simulink model "realtime_controller"  (R2025b)
settings: Solver=FixedStepAuto  StartTime=0.0  StopTime=inf  FixedStep=0.01  MaxStep=0.0001  RelTol=1e-3
model workspace (MAT data in the model file):
  B = 3.5077e-06
  J = 3.2284e-06
  Kt = 0.0274
  L = 2.75e-06
  Px_LUT = [72.8945083618 76.6020507812 80.0916442871 83.3246154785 86.26612854 88.8862457275 91.1605911255 93.0707244873 94.6042098999 95.7543792725 96.5199050903 96.9042816162 96.9152145386 96.5639724731 95.8647842407 94.8342666626 93.4909515381 91.8547897339 89.9468231201 87.7888336182 85.4030838013 82.8120956421 80.0384292603 77.1045608521 74.0327148438 70.8447647095 67.5620803833 64.2054595947 60.7950210571 57.3501052856 53.8891906738 50.4297790527 46.9883308411 43.5801582336 40.2193336487 36.9186134338 33.6893348694 30.5413703918 27.483045578 24.5211086273 21.6607170105 18.9054584503 16.2574234009 13.7173147202 11.2846326828 8.95790672302 6.73498630524 4.61337375641 2.59057831764 0.664467632771 -1.16641640663 -2.90260267258 -4.54352331161 -6.08744049072 -7.53147363663 -8.87170600891 -10.1033649445 -11.22103405 -12.2188882828 -13.090924263 -13.8311738968 -14.4338855743 -14.8936719894 -15.2056322098 -15.3654279709 -15.3693389893 -15.2142906189 -14.8978567123 -14.4182472229 -13.7742786407 -12.9653301239 -11.9912958145 -10.8525152206 -9.54971599579 -8.08393192291 -6.45643568039 -4.66865777969 -2.72211909294 -0.61836206913 1.64110088348 4.05482435226 6.6214389801 9.33963012695 12.208067894 15.2252807617 18.3894691467 21.6982364655 25.1482276917 28.734703064 32.4510154724 36.2880249023 40.2335128784 44.2715797424 48.3821792603 52.5407600403 56.7181930542 60.8809700012 64.9917602539 69.0102767944 72.8945083618]
  Py_LUT = [145.51965332 149.831832886 154.01940918 158.062957764 161.947036743 165.659683228 169.191879272 172.536972046 175.689926147 178.646850586 181.404403687 183.959472656 186.308914185 188.44934082 190.377151489 192.088546753 193.57951355 194.84602356 195.884170532 196.690216064 197.260864258 197.593276978 197.685287476 197.535476685 197.143264771 196.509063721 195.634277344 194.521408081 193.174133301 191.597320557 189.797027588 187.78062439 185.556686401 183.135070801 180.526931763 177.74458313 174.801589966 171.712585449 168.493286133 165.160308838 161.731033325 158.223480225 154.655960083 151.046920776 147.414581299 143.776626587 140.149795532 136.549667358 132.990280151 129.483917236 126.041030884 122.670181274 119.378143311 116.170150757 113.050140381 110.021156311 107.085639954 104.245857239 101.504173279 98.8633117676 96.3265914917 93.8980255127 91.5824508667 89.3855133057 87.3137207031 85.3743896484 83.5755691528 81.925994873 80.4349822998 79.1123504639 77.9683151245 77.013381958 76.2582168579 75.7135772705 75.3901138306 75.2982940674 75.4482421875 75.8495407104 76.5110855103 77.4408798218 78.6457595825 80.1312026978 81.9009857178 83.9569168091 86.2984542847 88.922416687 91.8225784302 94.9893722534 98.4095993042 102.066230774 105.938323975 110.001068115 114.226104736 118.581939697 123.034675598 127.548919678 132.088790894 136.61907959 141.106292725 145.51965332]
  R = 4
  Ts = 0.01
  a = 1
  theta2_LUT = [0 0.0634665191174 0.126933038235 0.190399557352 0.253866076469 0.317332595587 0.380799114704 0.444265633821 0.507732152939 0.571198642254 0.634665191174 0.698131680489 0.761598229408 0.825064718723 0.888531267643 0.951997756958 1.01546430588 1.0789308548 1.14239728451 1.20586383343 1.26933038235 1.33279693127 1.39626336098 1.4597299099 1.52319645882 1.58666300774 1.65012943745 1.71359598637 1.77706253529 1.84052908421 1.90399551392 1.96746206284 2.03092861176 2.09439516068 2.15786170959 2.2213280201 2.28479456902 2.34826111794 2.41172766685 2.47519421577 2.53866076469 2.60212731361 2.66559386253 2.72906017303 2.79252672195 2.85599327087 2.91945981979 2.98292636871 3.04639291763 3.10985946655 3.17332601547 3.23679232597 3.30025887489 3.36372542381 3.42719197273 3.49065852165 3.55412507057 3.61759161949 3.68105816841 3.74452447891 3.80799102783 3.87145757675 3.93492412567 3.99839067459 4.06185722351 4.12532377243 4.18879032135 4.25225687027 4.31572341919 4.37918996811 4.44265604019 4.50612258911 4.56958913803 4.63305568695 4.69652223587 4.75998878479 4.82345533371 4.88692188263 4.95038843155 5.01385498047 5.07732152939 5.14078807831 5.20425462723 5.26772117615 5.33118772507 5.39465427399 5.45812034607 5.52158689499 5.58505344391 5.64851999283 5.71198654175 5.77545309067 5.83891963959 5.90238618851 5.96585273743 6.02931928635 6.09278583527 6.15625238419 6.21971893311 6.28318548203]
undefined symbols (not defined in the file or in its folder): ControlMode, f
libraries: svdutilitieslib x5, arduinolib x5, slpidlib x2, instrumentlib x2, simulink x1, arduinosensorlib x1
settings Model: ExtModeTrigDuration=2  Creator=msmca  LastModifiedBy=msmca
settings SolverCC: AutoInsertRateTranBlk=on
settings DataIOCC: ReturnWorkspaceOutputs=off
settings OptimizationCC: DefaultParameterBehavior=Inlined  EnhancedBackFolding=on  PassReuseOutputArgsAs=Individual arguments  ZeroExternalMemoryAtStartup=off  ZeroInternalMemoryAtStartup=off  MaxStackSize=64  OptimizeBlockOrder=speed  DifferentSizesBufferReuse=on  OptimizationCustomize=off  EfficientTunableParamExpr=on
settings DebuggingCC: ParameterTunabilityLossMsg=error
settings HardwareCC: ProdBitPerInt=16.0  ProdBitPerPointer=16.0  ProdBitPerSizeT=16.0  ProdBitPerPtrDiffT=16.0  ProdLargestAtomicFloat=None  ProdWordSize=8.0  ProdHWDeviceType=Atmel->AVR
settings SFSimCC: MATLABDynamicMemAlloc=off
settings RTWCC: SystemTargetFile=ert.tlc  HardwareBoard=Arduino Uno  TemplateMakefile=ert_default_tmf  Toolchain=Arduino AVR  BuildConfiguration=Faster Runs  Description=Embedded Coder
settings CodeAppCC: ForceParamTrailComments=on  IgnoreCustomStorageClasses=off  OperatorAnnotations=on  SimulinkDataObjDesc=on  SFDataObjDesc=on  InsertBlockDesc=on
settings ERTTargetCC: ExtModeTransport=3.0  ExtModeStaticAlloc=on  ExtModeAutomaticAllocSize=off  ExtModeStaticAllocSize=250.0  ExtModeMexFile=ext_xcp  ExtModeIntrfLevel=Level2 - Open  InlinedParameterPlacement=Hierarchical  SupportContinuousTime=on  SupportVariableSizeSignals=on

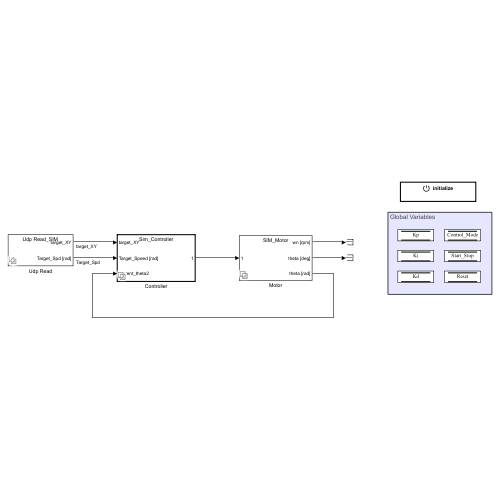
[thumbnail: Simulink's stored preview of the top-level diagram]
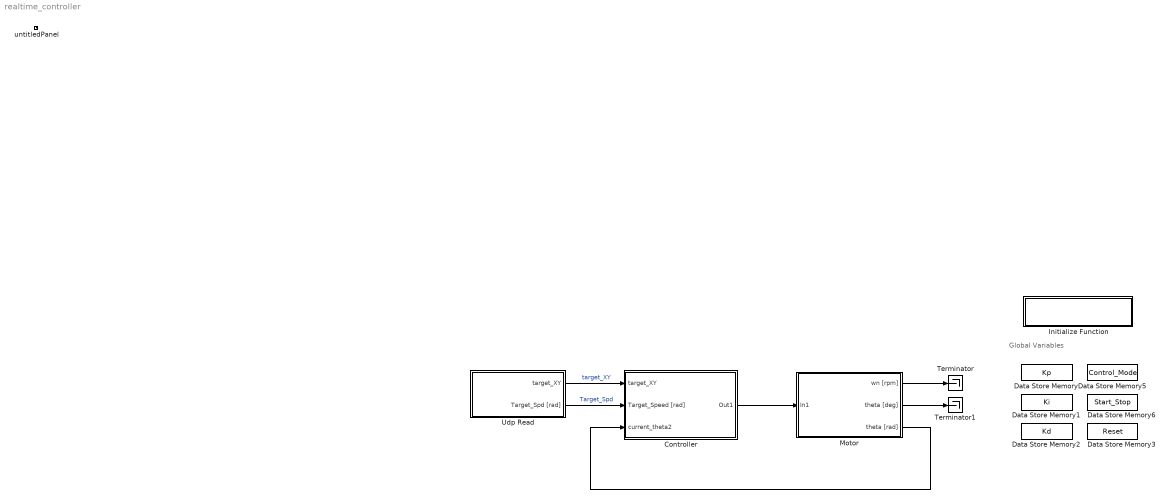
== system realtime_controller ==
  note: Global Variables
  Controller : Subsystem  TreatAsAtomicUnit=on  Variant=on  VariantControlMode=sim codegen switching  VariantControl=Controller  EmptyChoice=on
  Data Store Memory : DataStoreMemory  DataStoreName=Kp  WriteAfterWriteMsg=warning  ShowAdditionalParam=off
  Data Store Memory1 : DataStoreMemory  DataStoreName=Ki  WriteAfterWriteMsg=warning  ShowAdditionalParam=off
  Data Store Memory2 : DataStoreMemory  DataStoreName=Kd  WriteAfterWriteMsg=warning  ShowAdditionalParam=off
  Data Store Memory3 : DataStoreMemory  DataStoreName=Reset  WriteAfterWriteMsg=warning  ShowAdditionalParam=off
  Data Store Memory5 : DataStoreMemory  DataStoreName=Control_Mode  WriteAfterWriteMsg=warning  ShowAdditionalParam=off
  Data Store Memory6 : DataStoreMemory  DataStoreName=Start_Stop  WriteAfterWriteMsg=warning  ShowAdditionalParam=off  OutDataTypeStr=uint8
  Initialize Function : Subsystem  TreatAsAtomicUnit=on
  Motor : Subsystem  Variant=on  VariantControlMode=sim codegen switching  EmptyChoice=on
  Terminator : Terminator
  Terminator1 : Terminator
  Udp Read : Subsystem  Variant=on  VariantControlMode=sim codegen switching  EmptyChoice=on
  untitledPanel : Subsystem  Tag=HiddenForWebPanel  IsWebBlockPanel=on
  wires:
  Controller/1(Out1) -> Motor/1(In1)
  Motor/1(wn [rpm]) -> Terminator/1
  Motor/2(theta [deg]) -> Terminator1/1
  Motor/3(theta [rad]) -> Controller/3(current_theta2)
  Udp Read/1(target_XY) -> Controller/1(target_XY)  "target_XY"
  Udp Read/2(Target_Spd [rad]) -> Controller/2(Target_Speed [rad])  "Target_Spd"

== system realtime_controller/Controller ==
  target_XY : Inport
  Target_Speed [rad] : Inport  Port=2
  current_theta2 : Inport  Port=3
  Codegen_Controller : Subsystem  TreatAsAtomicUnit=on  VariantControl=(codegen)
  Sim_Controller : Subsystem  TreatAsAtomicUnit=on  VariantControl=(sim)
  Out1 : Outport

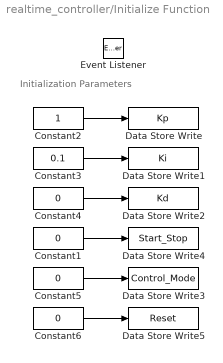
== system realtime_controller/Initialize Function ==
  note: Initialization Parameters
  Constant1 : Constant  Value=0  OutDataTypeStr=uint8
  Constant2 : Constant  OutDataTypeStr=single
  Constant3 : Constant  Value=0.1  OutDataTypeStr=single
  Constant4 : Constant  Value=0  OutDataTypeStr=single
  Constant5 : Constant  Value=0  OutDataTypeStr=uint8
  Constant6 : Constant  Value=0  OutDataTypeStr=uint8
  Data Store Write : DataStoreWrite  DataStoreName=Kp  IndexOptions=Index vector (dialog)  Indices=1  OutputSizes=1
  Data Store Write1 : DataStoreWrite  DataStoreName=Ki  IndexOptions=Index vector (dialog)  Indices=1  OutputSizes=1
  Data Store Write2 : DataStoreWrite  DataStoreName=Kd  IndexOptions=Index vector (dialog)  Indices=1  OutputSizes=1
  Data Store Write3 : DataStoreWrite  DataStoreName=Control_Mode  IndexOptions=Index vector (dialog)  Indices=1  OutputSizes=1
  Data Store Write4 : DataStoreWrite  DataStoreName=Start_Stop  IndexOptions=Index vector (dialog)  Indices=1  OutputSizes=1
  Data Store Write5 : DataStoreWrite  DataStoreName=Reset  IndexOptions=Index vector (dialog)  Indices=1  OutputSizes=1
  Event Listener : EventListener  DisableCoverage=on  EventName=reset
  wires:
  Constant2/1 -> Data Store Write/1
  Constant4/1 -> Data Store Write2/1
  Constant3/1 -> Data Store Write1/1
  Constant1/1 -> Data Store Write4/1
  Constant5/1 -> Data Store Write3/1
  Constant6/1 -> Data Store Write5/1

== system realtime_controller/Motor ==
  In1 : Inport
  Codgen_Motor : Subsystem  VariantControl=(codegen)
  SIM_Motor : Subsystem  VariantControl=(sim)
  wn [rpm] : Outport
  theta [deg] : Outport  Port=2
  theta [rad] : Outport  Port=3

== system realtime_controller/Udp Read ==
  Udp Read_Codegen : Subsystem  VariantControl=(codegen)
  Udp Read_SIM : Subsystem  VariantControl=(sim)
  target_XY : Outport
  Target_Spd [rad] : Outport  Port=2

== system realtime_controller/untitledPanel ==
  Display : DisplayBlock  Tag=HiddenForWebPanel  PanelInfo="{\"height\":69,\"left\":301,\"panelId\":\"panelId-5f5342a7-719f-4c1d-a791-b117091cac79\",\"top\":10,\"type\":\"panelChild\",\"version\":\"2019b\",\"width\":222,\"zIndex\":1500008}"  Transparency=1  GridColor=[0.502, 0.502, 0.502]
  Display1 : DisplayBlock  Tag=HiddenForWebPanel  PanelInfo="{\"height\":62,\"left\":196,\"panelId\":\"panelId-5f5342a7-719f-4c1d-a791-b117091cac79\",\"top\":15,\"type\":\"panelChild\",\"version\":\"2019b\",\"width\":94,\"zIndex\":1500004}"  Transparency=1  GridColor=[0.502, 0.502, 0.502]
  Display2 : DisplayBlock  Tag=HiddenForWebPanel  PanelInfo="{\"height\":57,\"left\":12,\"panelId\":\"panelId-5f5342a7-719f-4c1d-a791-b117091cac79\",\"top\":19,\"type\":\"panelChild\",\"version\":\"2019b\",\"width\":171,\"zIndex\":1500002}"  Format=Custom  Transparency=1  Layout=Fill available space  FormatString=%s  GridColor=[0.502, 0.502, 0.502]  ShowGrid=off
  Start/Stop : LampBlock  Tag=HiddenForWebPanel  PanelInfo="{\"height\":60,\"left\":550,\"panelId\":\"panelId-5f5342a7-719f-4c1d-a791-b117091cac79\",\"top\":20,\"type\":\"panelChild\",\"version\":\"2019b\",\"width\":65,\"zIndex\":1500006}"  DefaultColor=[192.0, 192.0, 192.0]
  panelInfo : PanelWebBlock  Tag=HiddenForWebPanel  PanelInfo="{\"compacted\":false,\"height\":86,\"isActiveTab\":true,\"left\":280,\"name\":\"Panel\",\"panelId\":\"panelId-5f5342a7-719f-4c1d-a791-b117091cac79\",\"tabIndex\":0,\"tabbedSetId\":\"tabbedSet4298033123\",\"top\":26,\"type\":\"panel\",\"version\":\"2019b\",\"visible\":true,\"width\":648,\"zIndex\":1500002}"  PanelSnapshot=<binary blob, 24248 chars, not shown>

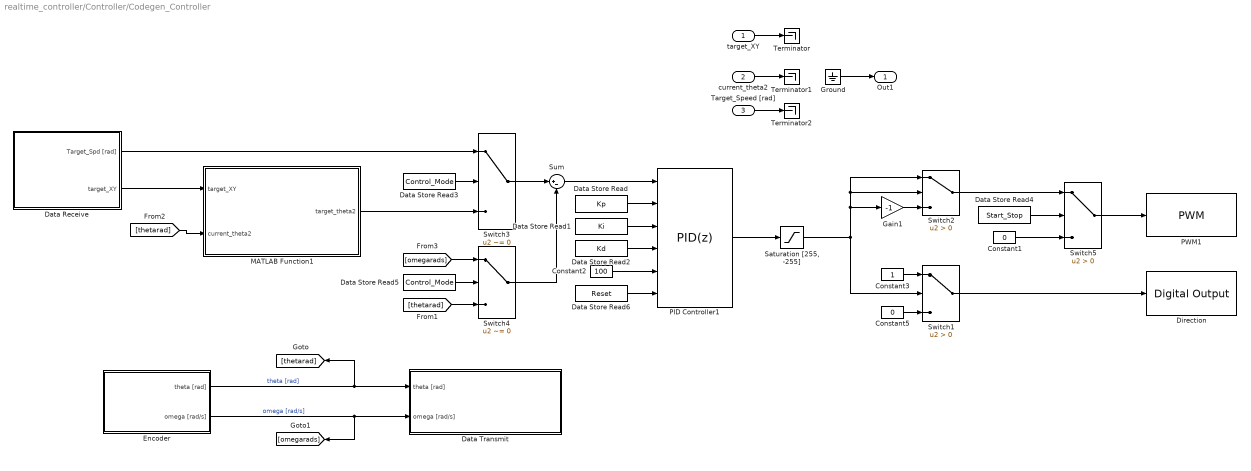
== system realtime_controller/Controller/Codegen_Controller ==
  target_XY : Inport
  current_theta2 : Inport  Port=2
  Target_Speed [rad] : Inport  Port=3
  Constant1 : Constant  Value=0  OutDataTypeStr=boolean
  Constant2 : Constant  Value=100  OutDataTypeStr=single
  Constant3 : Constant  OutDataTypeStr=boolean
  Constant5 : Constant  Value=0  OutDataTypeStr=boolean
  Data Receive : Subsystem
  Data Store Read : DataStoreRead  DataStoreName=Kp  IndexOptions=Index vector (dialog)  Indices=1  OutputSizes=1
  Data Store Read1 : DataStoreRead  DataStoreName=Ki  IndexOptions=Index vector (dialog)  Indices=1  OutputSizes=1
  Data Store Read2 : DataStoreRead  DataStoreName=Kd  IndexOptions=Index vector (dialog)  Indices=1  OutputSizes=1
  Data Store Read3 : DataStoreRead  DataStoreName=Control_Mode  IndexOptions=Index vector (dialog)  Indices=1  OutputSizes=1
  Data Store Read4 : DataStoreRead  DataStoreName=Start_Stop  IndexOptions=Index vector (dialog)  Indices=1  OutputSizes=1
  Data Store Read5 : DataStoreRead  DataStoreName=Control_Mode  IndexOptions=Index vector (dialog)  Indices=1  OutputSizes=1
  Data Store Read6 : DataStoreRead  DataStoreName=Reset  IndexOptions=Index vector (dialog)  Indices=1  OutputSizes=1
  Data Transmit : Subsystem
  Direction : arduinolib/Digital Output  pinNumber=9  Direction=output  blockPlatform=arduino
  Encoder : Subsystem
  Gain1 : Gain  Gain=-1
  Ground : Ground
  MATLAB Function1 : MATLAB Function  TreatAsAtomicUnit=on  VariantControl=CTRL_MODE == 1
      settings: RTWSystemCode=Inline
  PID Controller1 : slpidlib/PID Controller  Controller=PID  Form=Parallel  TimeDomain=Discrete-time  UseExternalTs=off  SampleTime=-1  IntegratorMethod=Forward Euler  FilterMethod=Forward Euler  ControllerParametersSource=external  P=236.110480401302  I=928.989984660749  UseKiTs=off  D=4.7957256427105  UseExternalDerivativeSource=off  N=1443.07789722776  UseFilter=on  TunerSelectOption=Transfer Function Based (PID Tuner App)  InitialConditionSource=internal  InitialConditionForIntegrator=0  InitialConditionForFilter=0  DifferentiatorICPrevScaledInput=0  ExternalReset=either  TrackingMode=off  Kt=1  LimitOutput=off  SatLimitsSource=internal  UpperSaturationLimit=24  LowerSaturationLimit=-24  LinearizeAsGain=on  AntiWindupMode=clamping  Kb=1  LimitIntegrator=on  UpperIntegratorSaturationLimit=35  LowerIntegratorSaturationLimit=-35  POutMin=[]  POutMax=[]  IOutMin=[]  IOutMax=[]  DOutMin=[]  DOutMax=[]  NOutMin=[]  NOutMax=[]  SumOutMin=[]  SumOutMax=[]  SaturationOutMin=[]  SaturationOutMax=[]  PParamMin=[]  PParamMax=[]  IParamMin=[]  IParamMax=[]  DParamMin=[]  DParamMax=[]  NParamMin=[]  NParamMax=[]  KbParamMin=[]  KbParamMax=[]  KtParamMin=[]  KtParamMax=[]  KbOutMin=[]  KbOutMax=[]  KtOutMin=[]  KtOutMax=[]  IntegratorOutMin=[]  IntegratorOutMax=[]  FilterOutMin=[]  FilterOutMax=[]  SumI1OutMin=[]  SumI1OutMax=[]  SumI2OutMin=[]  SumI2OutMax=[]  SumI3OutMin=[]  SumI3OutMax=[]  SumI4OutMin=[]  SumI4OutMax=[]  SumDOutMin=[]  SumDOutMax=[]  DifferentiatorOutMin=[]  DifferentiatorOutMax=[]  FilterDiffOutCoefMin=[]  FilterDiffOutCoefMax=[]  ReciprocalOutMin=[]  ReciprocalOutMax=[]  SumDenOutMin=[]  SumDenOutMax=[]  SumNumOutMin=[]  SumNumOutMax=[]  DivideOutMin=[]  DivideOutMax=[]  UdiffTsProdOutMin=[]  UdiffTsProdOutMax=[]  NTsProdOutMin=[]  NTsProdOutMax=[]  UintegralTsProdOutMin=[]  UintegralTsProdOutMax=[]  UngainTsProdOutMin=[]  UngainTsProdOutMax=[]  ClampingZeroOutDataTypeStr=Inherit: Inherit via back propagation  ClampingZeroOutMin=[]  ClampingZeroOutMax=[]  FilterDenConstantOutDataTypeStr=Inherit: Inherit via back propagation  FilterDenConstantOutMin=[]  FilterDenConstantOutMax=[]  PCopyOutDataTypeStr=Inherit: Inherit via back propagation  PCopyOutMin=[]  PCopyOutMax=[]  NCopyOutDataTypeStr=Inherit: Inherit via back propagation  NCopyOutMin=[]  NCopyOutMax=[]  IntegratorContinuousStateAttributes=''  IntegratorStateMustResolveToSignalObject=off  IntegratorRTWStateStorageClass=Auto  FilterContinuousStateAttributes=''  FilterStateMustResolveToSignalObject=off  FilterRTWStateStorageClass=Auto  ParallelPVariant=ExternalParameters  IdealPVariant=Disabled  IVariant=ExternalParameters  DVariant=ExternalParameters  IntegratorVariant=Discrete  SatVariant=Disabled  AWVariant=Passthrough  PCopyVariant=Disabled  TRVariant=Disabled  FdbkBlocksVariant=Forward  IdealPFdbkVariant=Disabled  SatFdbkVariant=Disabled  DerivativeFilterVariant=ForwardEulerFilter  NVariant=ExternalParameters  NCopyVariant=Disabled  FilterICVariant=InternalICsFilter  IntegratorICVariant=InternalICs  ExternalResetVariant=ExternalReset  TRSumVariant=Passthrough  SumFdbkVariant=Disabled  SumVariant=Sum_PID  TsampFilterVariant=InternalTs  TsampNgainVariant=Passthrough  TsampIntegralVariant=Disabled_SignalSpec  ExternalSaturationOutDataTypeStr=Inherit: Same as second input  DerivativeSourceVariant=ErrorSignal  PreIntVariant=InternalPreInt
  PWM1 : arduinolib/PWM  pinNumber=5  frequencyType=Default  desiredFrequency=490.2  achievableFrequency=490.2
  "Saturation [255, -255]" : Saturate  UpperLimit=254  LowerLimit=-254
  Sum : Sum  Inputs=|+-
  Switch1 : Switch  Criteria=u2 > Threshold  SaturateOnIntegerOverflow=off  InputSameDT=off
  Switch2 : Switch  Criteria=u2 > Threshold  OutDataTypeStr=single  SaturateOnIntegerOverflow=off  InputSameDT=off
  Switch3 : Switch  Criteria=u2 ~= 0  Threshold=0.5  SaturateOnIntegerOverflow=off  InputSameDT=off
  Switch4 : Switch  Criteria=u2 ~= 0  Threshold=0.5  SaturateOnIntegerOverflow=off  InputSameDT=off
  Switch5 : Switch  Criteria=u2 > Threshold  OutDataTypeStr=single  SaturateOnIntegerOverflow=off  InputSameDT=off
  Terminator : Terminator
  Terminator1 : Terminator
  Terminator2 : Terminator
  Out1 : Outport
  wires:
  PID Controller1/1 -> "Saturation [255, -255]"/1
  target_XY/1 -> Terminator/1
  current_theta2/1 -> Terminator1/1
  Data Receive/2(target_XY) -> MATLAB Function1/1(target_XY)
  Encoder/1(theta [rad]) -> Data Transmit/1(theta [rad]), [thetarad]  "theta [rad]"
  Encoder/2(omega [rad/s]) -> Data Transmit/2(omega [rad/s]), [omegarads]  "omega [rad/s]"
  Ground/1 -> Out1/1
  "Saturation [255, -255]"/1 -> Switch1/2, Gain1/1, Switch2/1, Switch2/2
  Gain1/1 -> Switch2/3
  Switch1/1 -> Direction/1
  Constant5/1 -> Switch1/3
  Constant3/1 -> Switch1/1
  Switch3/1 -> Sum/1
  Data Store Read3/1 -> Switch3/2
  MATLAB Function1/1(target_theta2) -> Switch3/3
  Switch4/1 -> Sum/2
  Data Store Read5/1 -> Switch4/2
  [thetarad] -> MATLAB Function1/2(current_theta2)
  [thetarad] -> Switch4/3
  [omegarads] -> Switch4/1
  Data Receive/1(Target_Spd [rad]) -> Switch3/1
  Switch5/1 -> PWM1/1
  Data Store Read4/1 -> Switch5/2
  Switch2/1 -> Switch5/1
  Constant1/1 -> Switch5/3
  Target_Speed [rad]/1 -> Terminator2/1
  Data Store Read/1 -> PID Controller1/2
  Data Store Read6/1 -> PID Controller1/6
  Data Store Read2/1 -> PID Controller1/4
  Data Store Read1/1 -> PID Controller1/3
  Sum/1 -> PID Controller1/1
  Constant2/1 -> PID Controller1/5

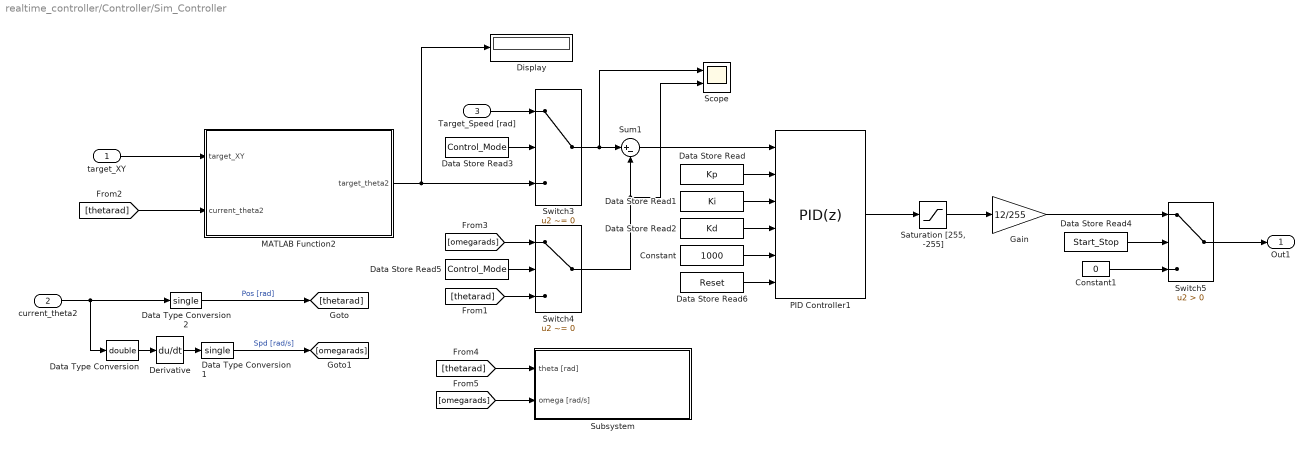
== system realtime_controller/Controller/Sim_Controller ==
  target_XY : Inport
  current_theta2 : Inport  Port=2
  Target_Speed [rad] : Inport  Port=3
  Constant : Constant  Value=1000  OutDataTypeStr=single
  Constant1 : Constant  Value=0  OutDataTypeStr=boolean
  Data Store Read : DataStoreRead  DataStoreName=Kp  IndexOptions=Index vector (dialog)  Indices=1  OutputSizes=1
  Data Store Read1 : DataStoreRead  DataStoreName=Ki  IndexOptions=Index vector (dialog)  Indices=1  OutputSizes=1
  Data Store Read2 : DataStoreRead  DataStoreName=Kd  IndexOptions=Index vector (dialog)  Indices=1  OutputSizes=1
  Data Store Read3 : DataStoreRead  DataStoreName=Control_Mode  IndexOptions=Index vector (dialog)  Indices=1  OutputSizes=1
  Data Store Read4 : DataStoreRead  DataStoreName=Start_Stop  IndexOptions=Index vector (dialog)  Indices=1  OutputSizes=1
  Data Store Read5 : DataStoreRead  DataStoreName=Control_Mode  IndexOptions=Index vector (dialog)  Indices=1  OutputSizes=1
  Data Store Read6 : DataStoreRead  DataStoreName=Reset  IndexOptions=Index vector (dialog)  Indices=1  OutputSizes=1
  Data Type Conversion : DataTypeConversion  OutDataTypeStr=double  SaturateOnIntegerOverflow=off  RndMeth=Floor
  Data Type Conversion1 : DataTypeConversion  OutDataTypeStr=single  SaturateOnIntegerOverflow=off  RndMeth=Floor
  Data Type Conversion2 : DataTypeConversion  OutDataTypeStr=single  SaturateOnIntegerOverflow=off  RndMeth=Floor
  Derivative : Derivative
  Display : Display
  Gain : Gain  Gain=12/255
  MATLAB Function2 : MATLAB Function  TreatAsAtomicUnit=on  VariantControl=CTRL_MODE == 1
  PID Controller1 : slpidlib/PID Controller  Controller=PID  Form=Parallel  TimeDomain=Discrete-time  UseExternalTs=off  SampleTime=-1  IntegratorMethod=Forward Euler  FilterMethod=Forward Euler  ControllerParametersSource=external  P=236.110480401302  I=928.989984660749  UseKiTs=off  D=4.7957256427105  UseExternalDerivativeSource=off  N=1443.07789722776  UseFilter=on  TunerSelectOption=Transfer Function Based (PID Tuner App)  InitialConditionSource=internal  InitialConditionForIntegrator=0  InitialConditionForFilter=0  DifferentiatorICPrevScaledInput=0  ExternalReset=either  TrackingMode=off  Kt=1  LimitOutput=off  SatLimitsSource=internal  UpperSaturationLimit=24  LowerSaturationLimit=-24  LinearizeAsGain=on  AntiWindupMode=clamping  Kb=1  LimitIntegrator=on  UpperIntegratorSaturationLimit=12  LowerIntegratorSaturationLimit=-12  POutMin=[]  POutMax=[]  IOutMin=[]  IOutMax=[]  DOutMin=[]  DOutMax=[]  NOutMin=[]  NOutMax=[]  SumOutMin=[]  SumOutMax=[]  SaturationOutMin=[]  SaturationOutMax=[]  PParamMin=[]  PParamMax=[]  IParamMin=[]  IParamMax=[]  DParamMin=[]  DParamMax=[]  NParamMin=[]  NParamMax=[]  KbParamMin=[]  KbParamMax=[]  KtParamMin=[]  KtParamMax=[]  KbOutMin=[]  KbOutMax=[]  KtOutMin=[]  KtOutMax=[]  IntegratorOutMin=[]  IntegratorOutMax=[]  FilterOutMin=[]  FilterOutMax=[]  SumI1OutMin=[]  SumI1OutMax=[]  SumI2OutMin=[]  SumI2OutMax=[]  SumI3OutMin=[]  SumI3OutMax=[]  SumI4OutMin=[]  SumI4OutMax=[]  SumDOutMin=[]  SumDOutMax=[]  DifferentiatorOutMin=[]  DifferentiatorOutMax=[]  FilterDiffOutCoefMin=[]  FilterDiffOutCoefMax=[]  ReciprocalOutMin=[]  ReciprocalOutMax=[]  SumDenOutMin=[]  SumDenOutMax=[]  SumNumOutMin=[]  SumNumOutMax=[]  DivideOutMin=[]  DivideOutMax=[]  UdiffTsProdOutMin=[]  UdiffTsProdOutMax=[]  NTsProdOutMin=[]  NTsProdOutMax=[]  UintegralTsProdOutMin=[]  UintegralTsProdOutMax=[]  UngainTsProdOutMin=[]  UngainTsProdOutMax=[]  ClampingZeroOutDataTypeStr=Inherit: Inherit via back propagation  ClampingZeroOutMin=[]  ClampingZeroOutMax=[]  FilterDenConstantOutDataTypeStr=Inherit: Inherit via back propagation  FilterDenConstantOutMin=[]  FilterDenConstantOutMax=[]  PCopyOutDataTypeStr=Inherit: Inherit via back propagation  PCopyOutMin=[]  PCopyOutMax=[]  NCopyOutDataTypeStr=Inherit: Inherit via back propagation  NCopyOutMin=[]  NCopyOutMax=[]  IntegratorContinuousStateAttributes=''  IntegratorStateMustResolveToSignalObject=off  IntegratorRTWStateStorageClass=Auto  FilterContinuousStateAttributes=''  FilterStateMustResolveToSignalObject=off  FilterRTWStateStorageClass=Auto  ParallelPVariant=ExternalParameters  IdealPVariant=Disabled  IVariant=ExternalParameters  DVariant=ExternalParameters  IntegratorVariant=Discrete  SatVariant=Disabled  AWVariant=Passthrough  PCopyVariant=Disabled  TRVariant=Disabled  FdbkBlocksVariant=Forward  IdealPFdbkVariant=Disabled  SatFdbkVariant=Disabled  DerivativeFilterVariant=ForwardEulerFilter  NVariant=ExternalParameters  NCopyVariant=Disabled  FilterICVariant=InternalICsFilter  IntegratorICVariant=InternalICs  ExternalResetVariant=ExternalReset  TRSumVariant=Passthrough  SumFdbkVariant=Disabled  SumVariant=Sum_PID  TsampFilterVariant=InternalTs  TsampNgainVariant=Passthrough  TsampIntegralVariant=Disabled_SignalSpec  ExternalSaturationOutDataTypeStr=Inherit: Same as second input  DerivativeSourceVariant=ErrorSignal  PreIntVariant=InternalPreInt
  "Saturation [255, -255]" : Saturate  UpperLimit=255  LowerLimit=-255
  Scope : Scope  NumInputPorts=2
      settings: ActiveDisplayYMinimum=-26.442962050437924  ActiveDisplayYMaximum=185.34457051753998
  Subsystem : Subsystem
  Sum1 : Sum  Inputs=|+-
  Switch3 : Switch  Criteria=u2 ~= 0  Threshold=0.5  SaturateOnIntegerOverflow=off  InputSameDT=off
  Switch4 : Switch  Criteria=u2 ~= 0  Threshold=0.5  SaturateOnIntegerOverflow=off  InputSameDT=off
  Switch5 : Switch  Criteria=u2 > Threshold  OutDataTypeStr=single  SaturateOnIntegerOverflow=off  InputSameDT=off
  Out1 : Outport
  wires:
  Data Store Read5/1 -> Switch4/2
  "Saturation [255, -255]"/1 -> Gain/1
  Data Store Read4/1 -> Switch5/2
  [thetarad] -> MATLAB Function2/2(current_theta2)
  Constant1/1 -> Switch5/3
  Data Store Read3/1 -> Switch3/2
  [omegarads] -> Switch4/1
  [thetarad] -> Switch4/3
  PID Controller1/1 -> "Saturation [255, -255]"/1
  Switch3/1 -> Scope/1, Sum1/1
  Switch4/1 -> Scope/2, Sum1/2
  Sum1/1 -> PID Controller1/1
  Switch5/1 -> Out1/1
  Gain/1 -> Switch5/1
  current_theta2/1 -> Data Type Conversion2/1, Data Type Conversion/1
  Derivative/1 -> Data Type Conversion1/1
  [thetarad] -> Subsystem/1(theta [rad])
  [omegarads] -> Subsystem/2(omega [rad/s])
  Data Type Conversion/1 -> Derivative/1
  Data Type Conversion1/1 -> [omegarads]  "Spd [rad/s]"
  MATLAB Function2/1(target_theta2) -> Display/1, Switch3/3
  Data Store Read/1 -> PID Controller1/2
  Data Store Read2/1 -> PID Controller1/4
  Constant/1 -> PID Controller1/5
  Data Type Conversion2/1 -> [thetarad]  "Pos [rad]"
  Target_Speed [rad]/1 -> Switch3/1
  target_XY/1 -> MATLAB Function2/1(target_XY)
  Data Store Read1/1 -> PID Controller1/3
  Data Store Read6/1 -> PID Controller1/6

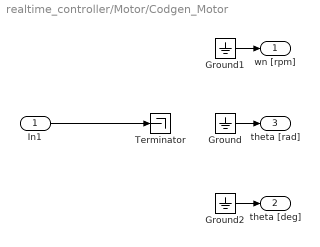
== system realtime_controller/Motor/Codgen_Motor ==
  In1 : Inport  OutDataTypeStr=single
  Ground : Ground
  Ground1 : Ground
  Ground2 : Ground
  Terminator : Terminator
  wn [rpm] : Outport  OutDataTypeStr=single
  theta [deg] : Outport  Port=2  OutDataTypeStr=single
  theta [rad] : Outport  Port=3  OutDataTypeStr=single
  wires:
  In1/1 -> Terminator/1
  Ground/1 -> theta [rad]/1
  Ground1/1 -> wn [rpm]/1
  Ground2/1 -> theta [deg]/1

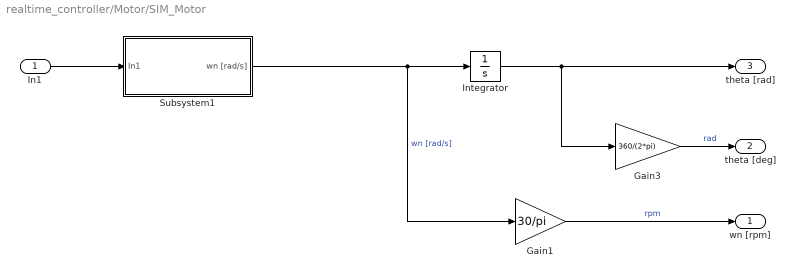
== system realtime_controller/Motor/SIM_Motor ==
  In1 : Inport
  Gain1 : Gain  Gain=30/pi  OutDataTypeStr=single
  Gain3 : Gain  Gain=360/(2*pi)  OutDataTypeStr=single
  Integrator : Integrator
  Subsystem1 : Subsystem
  wn [rpm] : Outport
  theta [deg] : Outport  Port=2
  theta [rad] : Outport  Port=3
  wires:
  Gain3/1 -> theta [deg]/1  "rad"
  Gain1/1 -> wn [rpm]/1  "rpm"
  In1/1 -> Subsystem1/1(In1)
  Integrator/1 -> theta [rad]/1, Gain3/1
  Subsystem1/1(wn [rad/s]) -> Integrator/1, Gain1/1  "wn [rad/s]"

== system realtime_controller/Udp Read/Udp Read_Codegen ==
  Ground : Ground
  Ground1 : Ground
  target_XY : Outport  OutDataTypeStr=single
  Target_Spd [rad] : Outport  Port=2  OutDataTypeStr=single
  wires:
  Ground/1 -> target_XY/1
  Ground1/1 -> Target_Spd [rad]/1

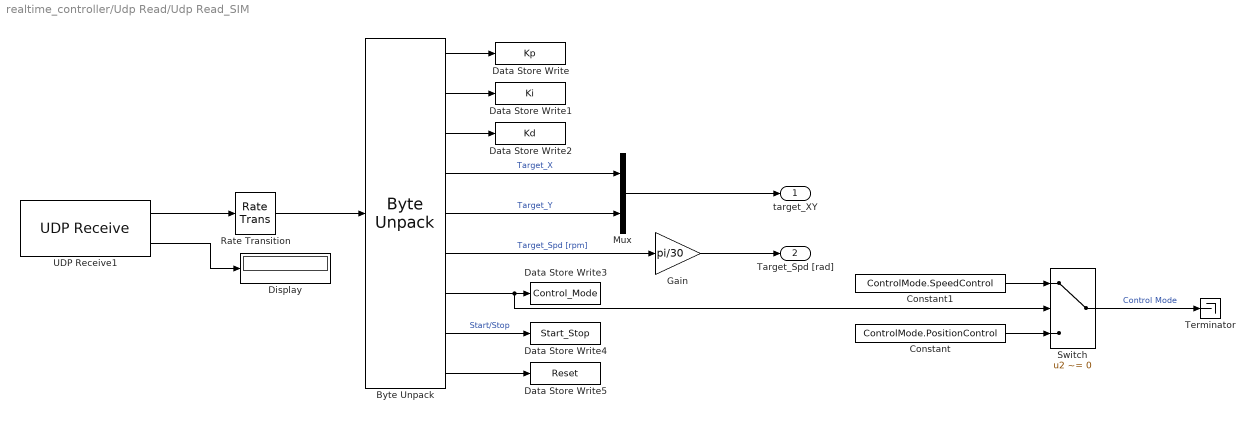
== system realtime_controller/Udp Read/Udp Read_SIM ==
  Byte Unpack : svdutilitieslib/Byte Unpack  dimensions={1, 1, 1, 1, 1, 1, 1, 1, 1}  datatypes={'single' 'single' 'single' 'single' 'single' 'single' 'uint8' 'uint8' 'uint8'}  byteAlign=1  blockPlatform=arduinoert
  Constant : Constant  Value=ControlMode.PositionControl
  Constant1 : Constant  Value=ControlMode.SpeedControl
  Data Store Write : DataStoreWrite  DataStoreName=Kp  IndexOptions=Index vector (dialog)  Indices=1  OutputSizes=1
  Data Store Write1 : DataStoreWrite  DataStoreName=Ki  IndexOptions=Index vector (dialog)  Indices=1  OutputSizes=1
  Data Store Write2 : DataStoreWrite  DataStoreName=Kd  IndexOptions=Index vector (dialog)  Indices=1  OutputSizes=1
  Data Store Write3 : DataStoreWrite  DataStoreName=Control_Mode  IndexOptions=Index vector (dialog)  Indices=1  OutputSizes=1
  Data Store Write4 : DataStoreWrite  DataStoreName=Start_Stop  IndexOptions=Index vector (dialog)  Indices=1  OutputSizes=1
  Data Store Write5 : DataStoreWrite  DataStoreName=Reset  IndexOptions=Index vector (dialog)  Indices=1  OutputSizes=1
  Display : Display
  Gain : Gain  Gain=pi/30
  Mux : Mux  Inputs=2
  Rate Transition : RateTransition  OutPortSampleTime=0.05
  Switch : Switch  Criteria=u2 ~= 0  Threshold=0.5  SaturateOnIntegerOverflow=off  InputSameDT=off
      settings: LockScale=on
  Terminator : Terminator
  UDP Receive1 : instrumentlib/UDP Receive  LocalAddress=0.0.0.0  LocalPort=5004  EnablePortSharing=off  Host=127.0.0.1  Port=5005  GetLatestData=on  DataSize=27  DataType=uint8  ASCIIFormatting=%f,  Terminator=LF  CustomTerminator=10  ByteOrder=big-endian  EnableBlockingMode=off  Timeout=10  SampleTime=0.001  SimulateUsing=Interpreted execution
  target_XY : Outport
  Target_Spd [rad] : Outport  Port=2
  wires:
  Byte Unpack/1 -> Data Store Write/1
  Mux/1 -> target_XY/1
  Byte Unpack/6 -> Gain/1  "Target_Spd [rpm]"
  Byte Unpack/8 -> Data Store Write4/1  "Start/Stop"
  Byte Unpack/5 -> Mux/2  "Target_Y"
  Byte Unpack/7 -> Switch/2, Data Store Write3/1
  Byte Unpack/4 -> Mux/1  "Target_X"
  UDP Receive1/2 -> Display/1
  Constant1/1 -> Switch/1
  Constant/1 -> Switch/3
  Switch/1 -> Terminator/1  "Control Mode"
  UDP Receive1/1 -> Rate Transition/1
  Byte Unpack/3 -> Data Store Write2/1
  Byte Unpack/2 -> Data Store Write1/1
  Rate Transition/1 -> Byte Unpack/1
  Gain/1 -> Target_Spd [rad]/1
  Byte Unpack/9 -> Data Store Write5/1

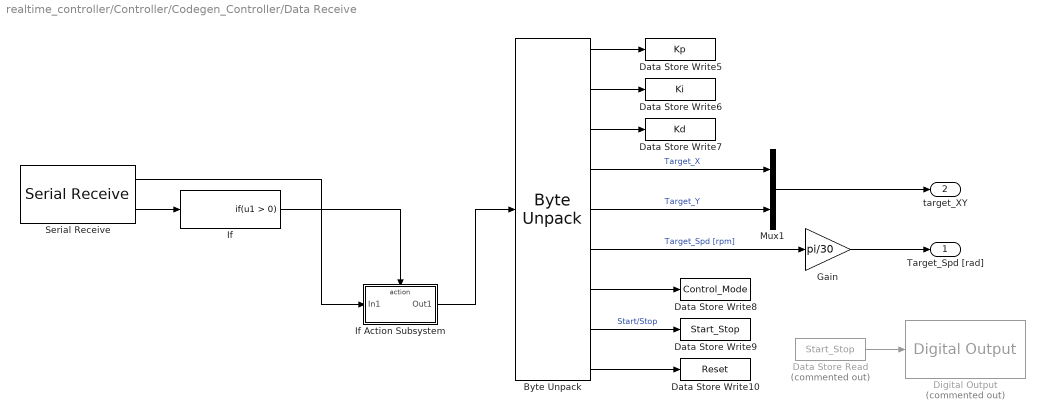
== system realtime_controller/Controller/Codegen_Controller/Data Receive ==
  Byte Unpack : svdutilitieslib/Byte Unpack  dimensions={1, 1, 1, 1, 1, 1, 1, 1, 1}  datatypes={'single' 'single' 'single' 'single' 'single' 'single' 'uint8' 'uint8' 'uint8'}  byteAlign=1  blockPlatform=arduinoert
  Data Store Read : DataStoreRead  Commented=on  DataStoreName=Start_Stop  IndexOptions=Index vector (dialog)  Indices=1  OutputSizes=1
  Data Store Write10 : DataStoreWrite  DataStoreName=Reset  IndexOptions=Index vector (dialog)  Indices=1  OutputSizes=1
  Data Store Write5 : DataStoreWrite  DataStoreName=Kp  IndexOptions=Index vector (dialog)  Indices=1  OutputSizes=1
  Data Store Write6 : DataStoreWrite  DataStoreName=Ki  IndexOptions=Index vector (dialog)  Indices=1  OutputSizes=1
  Data Store Write7 : DataStoreWrite  DataStoreName=Kd  IndexOptions=Index vector (dialog)  Indices=1  OutputSizes=1
  Data Store Write8 : DataStoreWrite  DataStoreName=Control_Mode  IndexOptions=Index vector (dialog)  Indices=1  OutputSizes=1
  Data Store Write9 : DataStoreWrite  DataStoreName=Start_Stop  IndexOptions=Index vector (dialog)  Indices=1  OutputSizes=1
  Digital Output : arduinolib/Digital Output  Commented=on  pinNumber=13  Direction=output  blockPlatform=arduino
  Gain : Gain  Gain=pi/30
  If : If  ShowElse=off
  If Action Subsystem : Subsystem  TreatAsAtomicUnit=on
  Mux1 : Mux  Inputs=2
  Serial Receive : arduinolib/Serial Receive  portNumber=0  DataType=uint8  blockPlatform=ARDUINO  TimeOut=0  MaxDataLength=10  isARMArch=off  DataLengthOption=Length via dialog  Datalength=27  Header=[170]  Terminator=[85]  SampleTime=0.05  ShowOutStatus=on
  Target_Spd [rad] : Outport
  target_XY : Outport  Port=2
  wires:
  Byte Unpack/4 -> Mux1/1  "Target_X"
  Gain/1 -> Target_Spd [rad]/1
  Mux1/1 -> target_XY/1
  Byte Unpack/2 -> Data Store Write6/1
  Byte Unpack/8 -> Data Store Write9/1  "Start/Stop"
  Byte Unpack/1 -> Data Store Write5/1
  Byte Unpack/5 -> Mux1/2  "Target_Y"
  Byte Unpack/6 -> Gain/1  "Target_Spd [rpm]"
  Byte Unpack/9 -> Data Store Write10/1
  Byte Unpack/7 -> Data Store Write8/1
  Byte Unpack/3 -> Data Store Write7/1
  Data Store Read/1 -> Digital Output/1
  Serial Receive/2 -> If/1
  If/1 -> If Action Subsystem/Action
  Serial Receive/1 -> If Action Subsystem/1(In1)
  If Action Subsystem/1(Out1) -> Byte Unpack/1

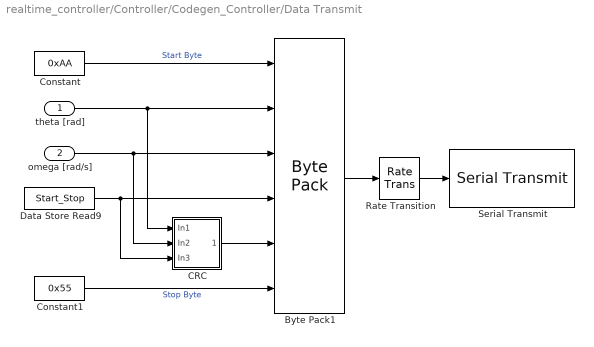
== system realtime_controller/Controller/Codegen_Controller/Data Transmit ==
  theta [rad] : Inport
  omega [rad/s] : Inport  Port=2
  Byte Pack1 : svdutilitieslib/Byte Pack  maskPackedDataType=uint8  datatypes={'uint8' 'single' 'single' 'uint8' 'uint8' 'uint8'}  byteAlign=1  blockPlatform=arduinoert
  CRC : Subsystem
  Constant : Constant  Value=0xAA  OutDataTypeStr=uint8
  Constant1 : Constant  Value=0x55  OutDataTypeStr=uint8
  Data Store Read9 : DataStoreRead  DataStoreName=Start_Stop  IndexOptions=Index vector (dialog)  Indices=1  OutputSizes=1
  Rate Transition : RateTransition  OutPortSampleTime=0.05
  Serial Transmit : arduinolib/Serial Transmit  portNumber=0  sendmode=write  sendformat=Decimal  floatprecision=2  header=[]  terminator=[]  blockPlatform=ARDUINO
  wires:
  Byte Pack1/1 -> Rate Transition/1
  Rate Transition/1 -> Serial Transmit/1
  theta [rad]/1 -> CRC/1(In1), Byte Pack1/2
  omega [rad/s]/1 -> CRC/2(In2), Byte Pack1/3
  Data Store Read9/1 -> CRC/3(In3), Byte Pack1/4
  Constant/1 -> Byte Pack1/1  "Start Byte"
  Constant1/1 -> Byte Pack1/6  "Stop Byte"
  CRC/1(CRC) -> Byte Pack1/5

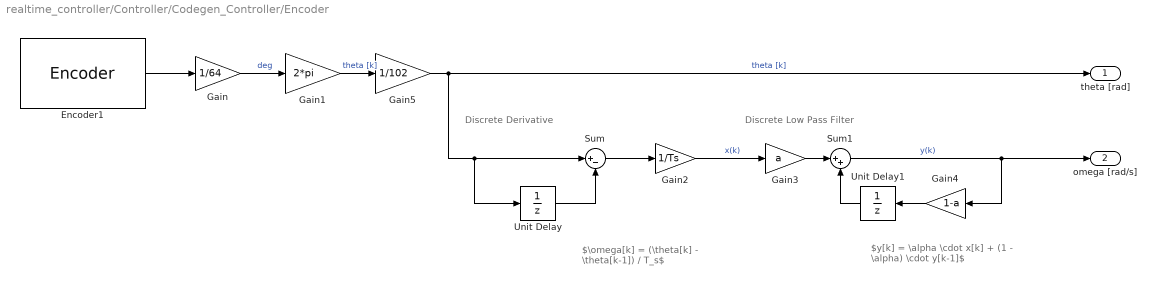
== system realtime_controller/Controller/Codegen_Controller/Encoder ==
  note: Discrete Low Pass Filter
  note: $y[k] = \alpha \cdot x[k] + (1 - \alpha) \cdot y[k-1]$
  note: $\omega[k] = (\theta[k] - \theta[k-1]) / T_s$
  note: Discrete Derivative
  Encoder1 : arduinosensorlib/Encoder  InputA=2  InputB=3  Mode=No reset  SampleTime=-1
  Gain : Gain  Gain=1/64  ParamDataTypeStr=single
  Gain1 : Gain  Gain=2*pi
  Gain2 : Gain  Gain=1/Ts
  Gain3 : Gain  Gain=a
  Gain4 : Gain  Gain=1-a
  Gain5 : Gain  Gain=1/102
  Sum : Sum  Inputs=|+-
  Sum1 : Sum  Inputs=|++
  Unit Delay : UnitDelay  SampleTime=Ts  HasFrameUpgradeWarning=on
  Unit Delay1 : UnitDelay  SampleTime=Ts  HasFrameUpgradeWarning=on
  theta [rad] : Outport
  omega [rad/s] : Outport  Port=2
  wires:
  Encoder1/1 -> Gain/1
  Gain/1 -> Gain1/1  "deg"
  Gain1/1 -> Gain5/1  "theta [k]"
  Sum/1 -> Gain2/1
  Unit Delay/1 -> Sum/2
  Gain2/1 -> Gain3/1  "x(k)"
  Gain3/1 -> Sum1/1
  Unit Delay1/1 -> Sum1/2
  Sum1/1 -> omega [rad/s]/1, Gain4/1  "y(k)"
  Gain4/1 -> Unit Delay1/1
  Gain5/1 -> Unit Delay/1, Sum/1, theta [rad]/1  "theta [k]"

== system realtime_controller/Controller/Sim_Controller/Subsystem ==
  theta [rad] : Inport
  omega [rad/s] : Inport  Port=2
  Byte Pack : svdutilitieslib/Byte Pack  maskPackedDataType=uint8  datatypes="{'single' 'single'  'uint8'}"  byteAlign=1  blockPlatform=arduinoert
      settings: LibrarySourceBlock=mcblib/Signal Management/Byte Pack
  Data Store Read9 : DataStoreRead  DataStoreName=Start_Stop  IndexOptions=Index vector (dialog)  Indices=1  OutputSizes=1
  Rate Transition : RateTransition  OutPortSampleTime=0.05
  UDP Send1 : instrumentlib/UDP Send  Host=127.0.0.1  Port=5005  LocalAddress=0.0.0.0  LocalPort=-1  EnablePortSharing=off  OutputDatagramPacketSize=512  ByteOrder=little-endian  EnableBlockingMode=on  SimulateUsing=Interpreted execution
  wires:
  Data Store Read9/1 -> Byte Pack/3
  omega [rad/s]/1 -> Byte Pack/2
  theta [rad]/1 -> Byte Pack/1
  Byte Pack/1 -> Rate Transition/1
  Rate Transition/1 -> UDP Send1/1

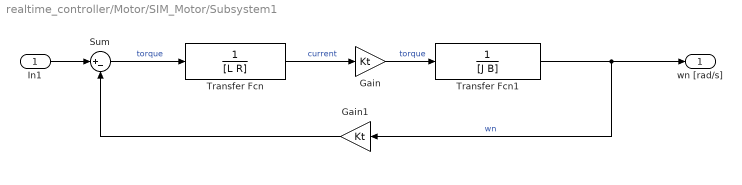
== system realtime_controller/Motor/SIM_Motor/Subsystem1 ==
  In1 : Inport
  Gain : Gain  Gain=Kt
  Gain1 : Gain  Gain=Kt
  Sum : Sum  Inputs=|+-
  Transfer Fcn : TransferFcn  Denominator=[L R]
  Transfer Fcn1 : TransferFcn  Denominator=[J B]
  wn [rad/s] : Outport
  wires:
  Transfer Fcn/1 -> Gain/1  "current"
  Gain1/1 -> Sum/2
  Transfer Fcn1/1 -> Gain1/1, wn [rad/s]/1  "wn"
  Gain/1 -> Transfer Fcn1/1  "torque"
  In1/1 -> Sum/1
  Sum/1 -> Transfer Fcn/1  "torque"

== system realtime_controller/Controller/Codegen_Controller/Data Receive/If Action Subsystem ==
  In1 : Inport
  Action Port : ActionPort  ActionPortLabel=if(u1 > 0)
  Out1 : Outport
  wires:
  In1/1 -> Out1/1

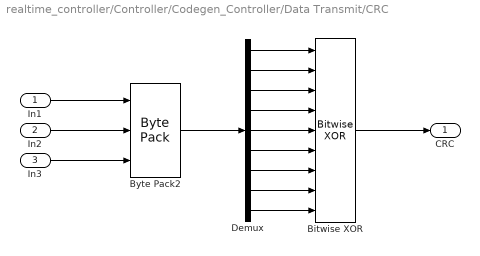
== system realtime_controller/Controller/Codegen_Controller/Data Transmit/CRC ==
  In1 : Inport
  In2 : Inport  Port=2
  In3 : Inport  Port=3
  Bitwise XOR : simulink/Logic and Bit Operations/Bitwise Operator  logicop=XOR  UseBitMask=off  NumInputPorts=9  BitMask=bin2dec('11011001')  BitMaskRealWorld=Stored Integer
      settings: LibrarySourceBlock=|
      | simulink/Quick Insert/Logic and Bit
      | Operations/Bitwise XOR
  Byte Pack2 : svdutilitieslib/Byte Pack  maskPackedDataType=uint8  datatypes={'single' 'single' 'uint8'}  byteAlign=1  blockPlatform=arduinoert
  Demux : Demux  Outputs=9
  CRC : Outport
  wires:
  Demux/4 -> Bitwise XOR/4
  Bitwise XOR/1 -> CRC/1
  Demux/3 -> Bitwise XOR/3
  Demux/6 -> Bitwise XOR/6
  Demux/8 -> Bitwise XOR/8
  Demux/5 -> Bitwise XOR/5
  Demux/2 -> Bitwise XOR/2
  Byte Pack2/1 -> Demux/1
  Demux/1 -> Bitwise XOR/1
  Demux/9 -> Bitwise XOR/9
  Demux/7 -> Bitwise XOR/7
  In2/1 -> Byte Pack2/2
  In1/1 -> Byte Pack2/1
  In3/1 -> Byte Pack2/3

== matlab function realtime_controller/Controller/Codegen_Controller/MATLAB Function1 ==
  settings: updateMethod=DISCRETE
  data: target_XY input; target_theta2 output; current_theta2 input; Px_LUT parameter single; Py_LUT parameter single; theta2_LUT parameter single
function target_theta2 = Arduino_Kinematics(target_XY, current_theta2, Px_LUT, Py_LUT, theta2_LUT)
    %#codegen
    X_ref = target_XY(1);
    Y_ref = target_XY(2);
% Başlangıç değerlerini ata (RAM dostu: sadece birkaç değişken)
    min_dist_sq = single(1e10); % Çok büyük bir sayı ile başla
    idx = int16(1);
% Vektörel işlem yerine tek tek dönerek en yakın noktayı bul
% Bu sayede RAM'de devasa geçici diziler oluşmaz
for i = 1:length(Px_LUT)
% Öklid mesafesinin karesini hesapla (Karekök alma, RAM ve CPU yorar)
        dist_sq = (Px_LUT(i) - X_ref)^2 + (Py_LUT(i) - Y_ref)^2;
if dist_sq < min_dist_sq
            min_dist_sq = dist_sq;
            idx = int16(i);
end
end
    raw_target_rad = theta2_LUT(idx);
% Phase Wrapping (En kısa yolu bul)
    delta_theta = mod(raw_target_rad - current_theta2 + pi, 2*pi) - pi;
    target_theta2 = current_theta2 + delta_theta;
end

== matlab function realtime_controller/Controller/Sim_Controller/MATLAB Function2 ==
  settings: updateMethod=DISCRETE
  data: target_XY input; target_theta2 output; current_theta2 input; Px_LUT parameter; Py_LUT parameter; theta2_LUT parameter
function target_theta2 = Arduino_Kinematics(target_XY, current_theta2, Px_LUT, Py_LUT, theta2_LUT)

%#codegen

% Arduino içinde gerçek zamanlı (real-time) çalışacak C kodu.

% LUT dizileri parametre olarak gelir (ROM/Flash belleğe gömülür).


X_ref = target_XY(1);

Y_ref = target_XY(2);


% Gelen X, Y hedefine en yakın açıyı bul (Nearest neighbor search)

dist_sq = (Px_LUT - X_ref).^2 + (Py_LUT - Y_ref).^2;

[~, idx] = min(dist_sq);

raw_target_rad = theta2_LUT(idx);


% Phase Wrapping (En kısa yolu bul)

delta_theta = mod(raw_target_rad - current_theta2 + pi, 2*pi) - pi;

target_theta2 = current_theta2 + delta_theta;

end
